simulink model "wielomian_zerujacy"  (R2018a)
settings: Solver=VariableStepAuto  StartTime=0.0  StopTime=100  RelTol=1e-3
values from neighbouring files (symbols this model uses):
  k = 1    [lms_z_eksperymentu.m]
undefined symbols (not defined in the file or in its folder): Ts, w
settings Model: Creator=klukomski  LastModifiedBy=klukomski

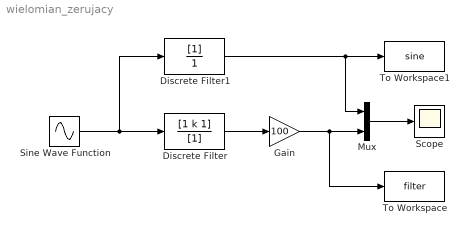
== system wielomian_zerujacy ==
  Discrete Filter : DiscreteFilter  Numerator=[1 k 1]  Denominator=[1]  SampleTime=Ts
  Discrete Filter1 : DiscreteFilter  Denominator=1  SampleTime=2*pi/(500*w*Ts)
  Gain : Gain  Gain=100
  Mux : Mux  Inputs=2
  Scope : Scope
  Sine Wave Function : Sin  Amplitude=5  Bias=10  Frequency=w*1.1  Phase=30  SampleTime=0
  To Workspace : ToWorkspace  VariableName=filter  SaveFormat=Timeseries  SampleTime=-1
  To Workspace1 : ToWorkspace  VariableName=sine  SaveFormat=Timeseries  SampleTime=-1
  wires:
  Sine Wave Function/1 -> Discrete Filter1/1, Discrete Filter/1
  Mux/1 -> Scope/1
  Discrete Filter1/1 -> Mux/1, To Workspace1/1
  Discrete Filter/1 -> Gain/1
  Gain/1 -> To Workspace/1, Mux/2
